simulink model "seat_heating_control"  (R2024b)
settings: Solver=FixedStepDiscrete  StartTime=0.0  StopTime=10.0  FixedStep=0.01  RelTol=1e-3
settings Model: Creator=nabilekhoury  LastModifiedBy=developer
settings SolverCC: AlgebraicLoopSolver=TrustRegion
settings DataIOCC: SaveFormat=StructureWithTime
settings OptimizationCC: DefaultParameterBehavior=Inlined  EnhancedBackFolding=on  MemcpyThreshold=640  PassReuseOutputArgsAs=Individual arguments  ZeroExternalMemoryAtStartup=off  ZeroInternalMemoryAtStartup=off  InitFltsAndDblsToZero=on  OptimizeBlockOrder=speed  DifferentSizesBufferReuse=on  OptimizationCustomize=off  EfficientTunableParamExpr=on
settings DebuggingCC: ParameterTunabilityLossMsg=error  UnconnectedInputMsg=warning  UnconnectedOutputMsg=warning  UnconnectedLineMsg=warning  ArithmeticOperatorsInVariantConditions=warning
settings ModelReferenceCC: EnableRefExpFcnMdlSchedulingChecks=on  ModelReferenceNumInstancesAllowed=Single
settings SFSimCC: MATLABDynamicMemAlloc=off  CustomCodeUndefinedFunction=UseInterfaceOnly
settings RTWCC: Description=Embedded Coder  SystemTargetFile=ert.tlc  GenCodeOnly=on  TemplateMakefile=ert_default_tmf  IncludeHyperlinkInReport=on  GPUComputeCapability=3.5
settings CodeAppCC: ForceParamTrailComments=on  IgnoreCustomStorageClasses=off  OperatorAnnotations=on  SimulinkDataObjDesc=on  SFDataObjDesc=on  InsertBlockDesc=on
settings ERTTargetCC: TargetLangStandard=C99 (ISO)  GenerateSampleERTMain=on  SupportAbsoluteTime=off  SupportNonFinite=off  SupportComplex=off  ERTCustomFileTemplate=example_file_process.tlc  DynamicArrayContainerType=coder::array

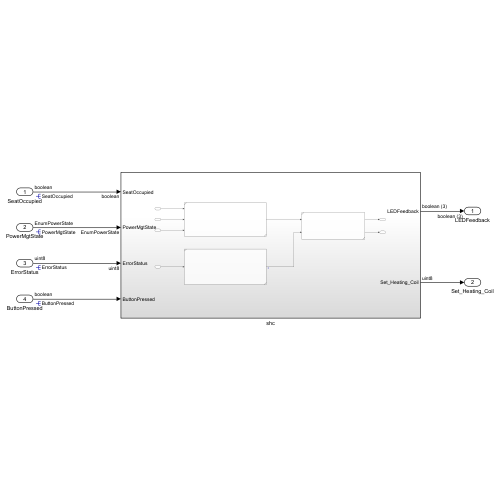
[thumbnail: Simulink's stored preview of the top-level diagram]
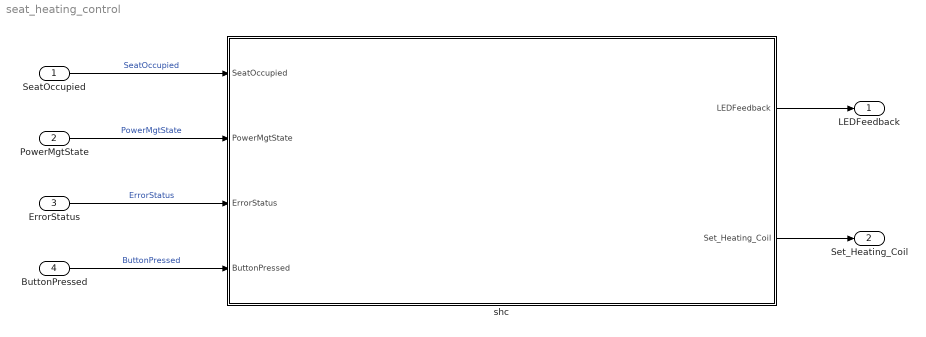
== system seat_heating_control ==
  SeatOccupied : Inport  OutDataTypeStr=boolean  PortDimensions=1
  PowerMgtState : Inport  Port=2  OutDataTypeStr=Enum: EnumPowerState  PortDimensions=1
  ErrorStatus : Inport  Port=3  OutDataTypeStr=uint8  PortDimensions=1
  ButtonPressed : Inport  Port=4
  shc : Subsystem
  LEDFeedback : Outport  OutDataTypeStr=boolean
  Set_Heating_Coil : Outport  Port=2
  wires:
  SeatOccupied/1 -> shc/1(SeatOccupied)  "SeatOccupied"
  PowerMgtState/1 -> shc/2(PowerMgtState)  "PowerMgtState"
  ErrorStatus/1 -> shc/3(ErrorStatus)  "ErrorStatus"
  ButtonPressed/1 -> shc/4(ButtonPressed)  "ButtonPressed"
  shc/2(Set_Heating_Coil) -> Set_Heating_Coil/1
  shc/1(LEDFeedback) -> LEDFeedback/1

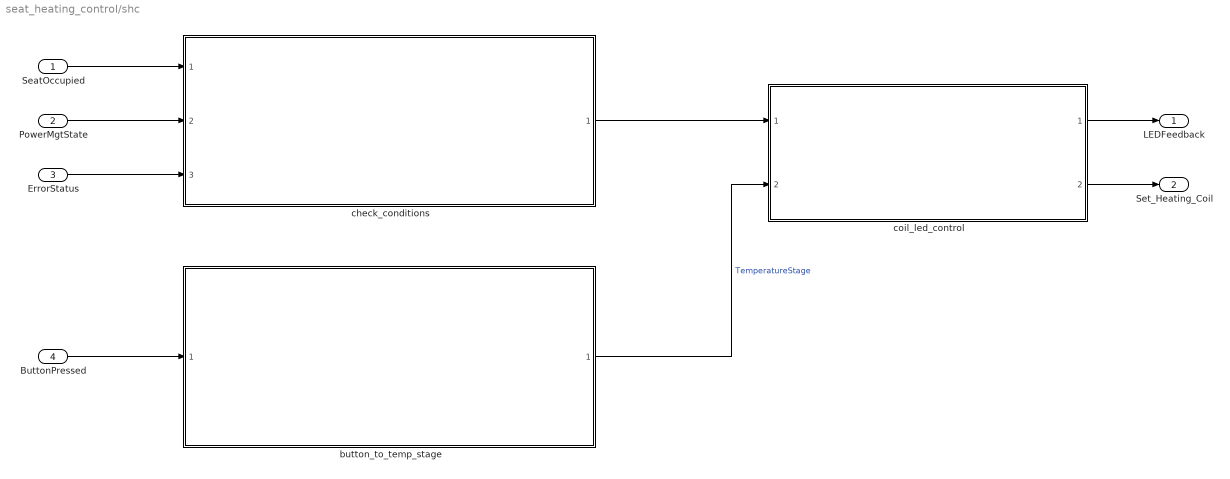
== system seat_heating_control/shc ==
  SeatOccupied : Inport  OutDataTypeStr=boolean  PortDimensions=1
  PowerMgtState : Inport  Port=2  OutDataTypeStr=Enum: EnumPowerState  PortDimensions=1
  ErrorStatus : Inport  Port=3  OutDataTypeStr=uint8  PortDimensions=1
  ButtonPressed : Inport  Port=4
  button_to_temp_stage : Subsystem  TreatAsAtomicUnit=on  RTWFcnName=button_to_temp_stage  ReferencedSubsystem=button_to_temp_stage
      settings: RTWSystemCode=Nonreusable function  RTWFcnNameOpts=User specified  RTWFileNameOpts=Use subsystem name
  check_conditions : Subsystem  TreatAsAtomicUnit=on  RTWFcnName=check_conditions  ReferencedSubsystem=check_conditions
      settings: RTWSystemCode=Nonreusable function  RTWFcnNameOpts=User specified  RTWFileNameOpts=Use subsystem name
  coil_led_control : Subsystem  TreatAsAtomicUnit=on  RTWFcnName=coil_led_control  ReferencedSubsystem=coil_led_control
      settings: RTWSystemCode=Nonreusable function  RTWFcnNameOpts=User specified  RTWFileNameOpts=Use subsystem name
  LEDFeedback : Outport  OutDataTypeStr=boolean
  Set_Heating_Coil : Outport  Port=2
  wires:
  check_conditions/1 -> coil_led_control/1
  ButtonPressed/1 -> button_to_temp_stage/1
  coil_led_control/2 -> Set_Heating_Coil/1
  PowerMgtState/1 -> check_conditions/2
  SeatOccupied/1 -> check_conditions/1
  button_to_temp_stage/1 -> coil_led_control/2  "TemperatureStage"
  ErrorStatus/1 -> check_conditions/3
  coil_led_control/1 -> LEDFeedback/1
